simulink model "mcb_microchip_pmsm_foc_sensorless_PIC32MK1024MCF"  (R2023b)
settings: Solver=FixedStepDiscrete  StartTime=0.0  StopTime=5  FixedStep=Ts  RelTol=1e-3  EnableMultiTasking=on
InitFcn:
  | mcb_microchip_pmsm_foc_sensorless_pic32mk_data
values from neighbouring files (symbols this model uses):
  PI_params = mcb.internal.SetControllerParameters(pmsm,inverter,PU_System,T_pwm,2*Ts,Ts_speed)    [mcb_microchip_pmsm_foc_sensorless_pic32mk_data.m]
  PU_System = mcb_SetPUSystem(pmsm,inverter)    [mcb_microchip_pmsm_foc_sensorless_pic32mk_data.m]
  PWM_frequency = 12e3    (= 12000)    [mcb_microchip_pmsm_foc_sensorless_pic32mk_data.m]
  Ts = T_pwm    (= 8.33333333333e-05)    [mcb_microchip_pmsm_foc_sensorless_pic32mk_data.m]
  Ts_motor = T_pwm    (= 8.33333333333e-05)    [mcb_microchip_pmsm_foc_sensorless_pic32mk_data.m]
  Ts_simulink = T_pwm    (= 8.33333333333e-05)    [mcb_microchip_pmsm_foc_sensorless_pic32mk_data.m]
  Ts_speed = 1e-3    (= 0.001)    [mcb_microchip_pmsm_foc_sensorless_pic32mk_data.m]
  Vd_Ref_openLoop_PU = 0.15    [mcb_microchip_pmsm_foc_sensorless_pic32mk_data.m]
undefined symbols (not defined in the file or in its folder): A0, A11, A4, AN24, AN9, B6, B9, C8, DiscIntNeverNeededParam, inverter, Pin, pmsm, Timer
libraries: simulink x16, MCHP_Blockset x12, mcbcontrolslib x10, slpidlib x3, mcbpositiondecoderlib x2, mcbplantlib x1, autolibpmsmexterior x1
(part 2 of 3)

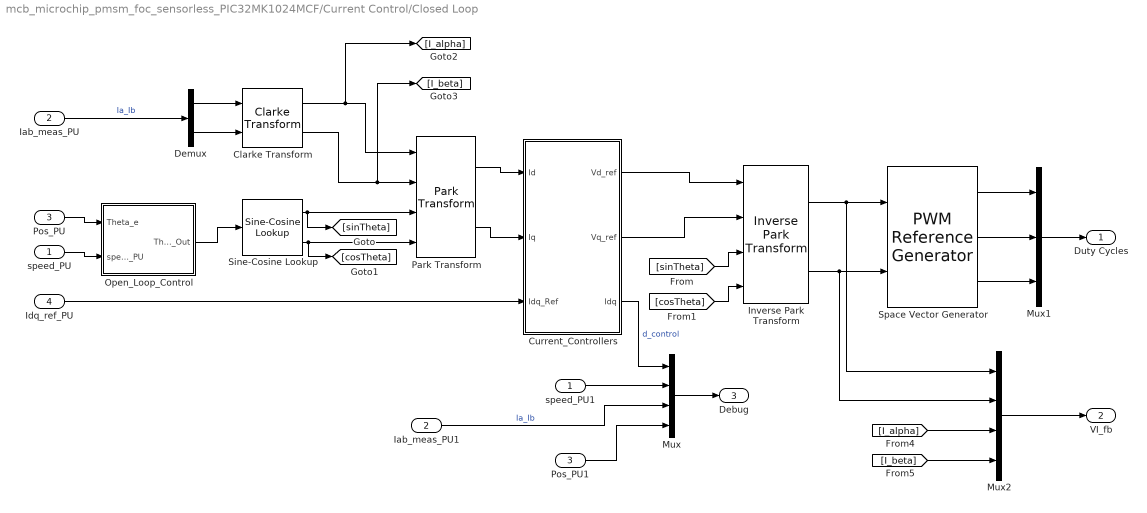
== system mcb_microchip_pmsm_foc_sensorless_PIC32MK1024MCF/Current Control/Closed Loop ==
  speed_PU : Inport
  Iab_meas_PU : Inport  Port=2
  Pos_PU : Inport  Port=3
  Idq_ref_PU : Inport  Port=4
  Clarke Transform : mcbcontrolslib/Clarke Transform  VariantControl=Variant2  PhaseInput=Two inputs  EnPowerInv=off
  Current_Controllers : Subsystem
  Demux : Demux  Outputs=2
  Iab_meas_PU1 : InportShadow  Port=2
  Inverse Park Transform : mcbcontrolslib/Inverse Park Transform  PhaseInput=Two inputs  AxisAlignment=D-axis  ThetaInput=Sine and Cosine electrical position  AngleInput=Per-unit  N_points=1024
  Mux : Mux
  Mux1 : Mux  Inputs=3
  Mux2 : Mux
  Open_Loop_Control : Subsystem
  Park Transform : mcbcontrolslib/Park Transform  PhaseInput=Two inputs  AxisAlignment=D-axis  ThetaInput=Sine and Cosine electrical position  AngleInput=Per-unit  N_points=1024
  Pos_PU1 : InportShadow  Port=3
  Sine-Cosine Lookup : mcbcontrolslib/Sine-Cosine Lookup  AngleInput=Per-unit  N_points=1024
  Space Vector Generator : mcbcontrolslib/PWM Reference Generator  inSignal=Valphabeta  modType=SVM: space vector modulation
  speed_PU1 : InportShadow
  Duty Cycles : Outport  VectorParamsAs1DForOutWhenUnconnected=off
  VI_fb : Outport  Port=2  VectorParamsAs1DForOutWhenUnconnected=off
  Debug : Outport  Port=3  VectorParamsAs1DForOutWhenUnconnected=off
  wires:
  Current_Controllers/1(Vd_ref) -> Inverse Park Transform/1
  [cosTheta] -> Inverse Park Transform/4
  [I_beta] -> Mux2/4
  Inverse Park Transform/2 -> Space Vector Generator/2, Mux2/2
  Inverse Park Transform/1 -> Space Vector Generator/1, Mux2/1
  [sinTheta] -> Inverse Park Transform/3
  Mux2/1 -> VI_fb/1
  Clarke Transform/1 -> [I_alpha], Park Transform/1
  Current_Controllers/2(Vq_ref) -> Inverse Park Transform/2
  Clarke Transform/2 -> [I_beta], Park Transform/2
  Sine-Cosine Lookup/1 -> [sinTheta], Park Transform/3
  [I_alpha] -> Mux2/3
  Space Vector Generator/1 -> Mux1/1
  Space Vector Generator/3 -> Mux1/3
  Mux1/1 -> Duty Cycles/1
  Sine-Cosine Lookup/2 -> Park Transform/4, [cosTheta]
  Space Vector Generator/2 -> Mux1/2
  Park Transform/1 -> Current_Controllers/1(Id)
  Park Transform/2 -> Current_Controllers/2(Iq)
  Demux/1 -> Clarke Transform/1
  Demux/2 -> Clarke Transform/2
  Iab_meas_PU/1 -> Demux/1  "Ia_Ib"
  Idq_ref_PU/1 -> Current_Controllers/3(Idq_Ref)
  Pos_PU/1 -> Open_Loop_Control/1(Theta_e)
  Open_Loop_Control/1(Theta_Out) -> Sine-Cosine Lookup/1
  speed_PU/1 -> Open_Loop_Control/2(speed_PU)
  speed_PU1/1 -> Mux/2
  Current_Controllers/3(Idq) -> Mux/1  "d_control"
  Mux/1 -> Debug/1
  Iab_meas_PU1/1 -> Mux/3  "Ia_Ib"
  Pos_PU1/1 -> Mux/4

== system mcb_microchip_pmsm_foc_sensorless_PIC32MK1024MCF/Current Control/HW Inputs ==
  Sim : Inport
  Sensor Driver Blocks (codegen) : Subsystem  VariantControl=(codegen)
  Sensor Driver Blocks (sim) : Subsystem  VariantControl=(sim)
  Iab_ADC : Outport

== system mcb_microchip_pmsm_foc_sensorless_PIC32MK1024MCF/Current Control/Input Scaling ==
  note: Current Measurements
  Iab_ADC : Inport
  VI_fb : Inport  Port=2
  Calculate Phase Currents : Subsystem
  Calculate position and speed : Subsystem
  speed_PU : Outport
  Iab_meas_PU : Outport  Port=2
  Pos_PU : Outport  Port=3
  wires:
  Calculate Phase Currents/1(Iab_meas_PU) -> Iab_meas_PU/1  "Iab_fb_PU"
  Iab_ADC/1 -> Calculate Phase Currents/1(Iab_ADC)
  Calculate position and speed/2(speed_PU) -> speed_PU/1
  Calculate position and speed/1(Pos_PU) -> Pos_PU/1
  VI_fb/1 -> Calculate position and speed/1(VI_fb)

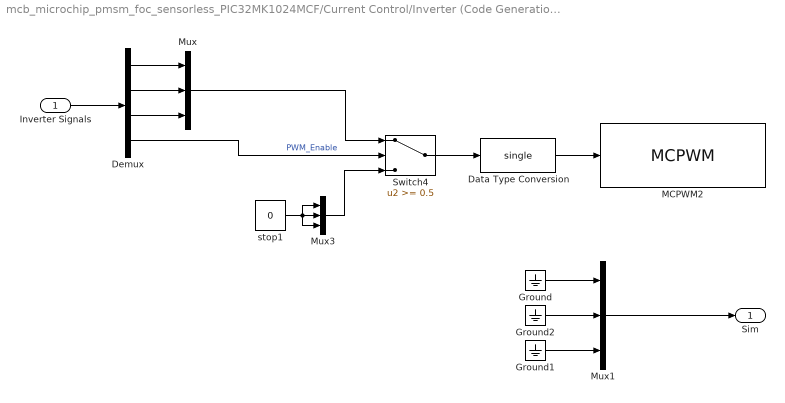
== system mcb_microchip_pmsm_foc_sensorless_PIC32MK1024MCF/Current Control/Inverter (Code Generation) ==
  Inverter Signals : Inport
  Data Type Conversion : DataTypeConversion  OutDataTypeStr=single  SaturateOnIntegerOverflow=off  RndMeth=Floor
  Demux : Demux
  Ground : Ground
  Ground1 : Ground
  Ground2 : Ground
  MCPWM2 : MCHP_Blockset/PWM IO/MCPWM  Priority=-2000  PWMx_ECAM_ITB=Independant - Center aligned - Symetric  PWMx_MTBS=Primary master timer  PWM_ClockResolution=Dynamic Options  PWM_ClockResolution_TXT=auto  MaxPeriod_s=Ts  InitPeriode_s=Ts  InitDutyCycleP_s=10e-6  InitDutyCycleS_s=10e-6  InitPhase_s=-1  SampleTime=Ts  S_INPUT=[-1]  S_INPUT_Size=[3]  S_OUTPUT=[]  S_OUTPUT_Size=[]  S_ListCustomDatatype=S.S_ListCustomDatatype={};  MCHP_USER_INTERRUPTS=0  evalin_ws=PWM1max=MCHP_Fun.Hex2num('40B3880000000000');PWM2max=MCHP_Fun.Hex2num('40B3880000000000');PWM3max=MCHP_Fun.Hex2num('40B3880000000000');  MCHP_PORT={PWMH1 }{PWMH1}32:4:B14;{PWMH2 }{PWMH2}32:4:B12;{PWMH3 }{PWMH3}32:4:B10;{PWML1}{PWML1}32:4:B15;{PWML2}{PWML2}32:4:B13;{PWML3}{PWML3}32:4:B11;{PWM FLT15}{FLT15}32:0:B4;  MCHP_MASTERLINK=mcb_microchip_pmsm_foc_sensorless_PIC32MK/Configurations/Microchip Master  MCHP_CRC=3937595  PWMx_PMOD=Complementary  PWM1_HL=PWMxH & PWMxL output enabled  PWM1_swap=off  PWM1H_pol=off  PWM1L_pol=off  PWM2_HL=PWMxH & PWMxL output enabled  PWM2_swap=off  PWM2H_pol=off  PWM2L_pol=off  PWM3_HL=PWMxH & PWMxL output enabled  PWM3_swap=off  PWM3H_pol=off  PWM3L_pol=off  PWM4_HL=not used  PWM4_swap=off  PWM4H_pol=off  PWM4L_pol=off  PWM5_HL=not used  PWM5_swap=off  PWM5H_pol=off  PWM5L_pol=off  PWM6_HL=not used  PWM6_swap=off  PWM6H_pol=off  PWM6L_pol=off  PWM7_HL=not used  PWM7_swap=off  PWM7H_pol=off  PWM7L_pol=off  PWM8_HL=not used  PWM8_swap=off  PWM8H_pol=off  PWM8L_pol=off  PWM9_HL=not used  PWM9_swap=off  PWM9H_pol=off  PWM9L_pol=off  PWM10_HL=not used  PWM10_swap=off  PWM10H_pol=off  PWM10L_pol=off  PWM11_HL=not used  PWM11_swap=off  PWM11H_pol=off  PWM11L_pol=off  PWM12_HL=not used  PWM12_swap=off  PWM12H_pol=off  PWM12L_pol=off  Init_SEVTCMP_SSEVTCMP=-1  Init_TRIGx_STRIGx_1=[1.8e-6 ,-1]  Init_TRIGx_STRIGx_2=[-1 -1]  Init_TRIGx_STRIGx_3=[-1 -1]  Init_TRIGx_STRIGx_4=[-1 -1]  Init_TRIGx_STRIGx_5=[-1 -1]  Init_TRIGx_STRIGx_6=[-1 -1]  Init_TRIGx_STRIGx_7=[-1 -1]  Init_TRIGx_STRIGx_8=[-1 -1]  Init_TRIGx_STRIGx_9=[-1 -1]  Init_TRIGx_STRIGx_10=[-1 -1]  Init_TRIGx_STRIGx_11=[-1 -1]  Init_TRIGx_STRIGx_12=[-1 -1]  TRIG_DualTriggerMode=Primary Trigger to ADC is independant  BlockInput_VectorScalar=Vectors (grouped by function)  BlockInput_Period=Not a block input  BlockInput_DutyCycle=a Floating Point input within range [-1 1]  BlockInput_PhaseShift=Not a block input  BlockInput_SEVTCMP=Not a block input  BlockInput_TRIGx=Not a block input  BlockInput_DeadTime=Not a block input  BlockOutput_FaultDisabled=off  BlockOutput_Fault=off  DTC=Positive dead time (ensure period of time with PWM_H and PWM_L disasserted)  FLTSRC1_DTCMP=Dynamic Options  FLTSRC1_DTCMP_TXT="FLT6 / E13 / Pin[42]  -  Active HIGH"  FLTSRC2_DTCMP=Dynamic Options  FLTSRC2_DTCMP_TXT="FLT6 / E13 / Pin[42]  -  Active LOW"  FLTSRC3_DTCMP=Dynamic Options  FLTSRC3_DTCMP_TXT="FLT8 / E15 / Pin[44]  -  Active LOW"  FLTSRC4_DTCMP=Dynamic Options  FLTSRC4_DTCMP_TXT="FLT3 / C2 / Pin[34]  -  Active HIGH"  FLTSRC5_DTCMP=Dynamic Options  FLTSRC5_DTCMP_TXT="FLT3 / C2 / Pin[34]  -  Active HIGH"  FLTSRC6_DTCMP=Dynamic Options  FLTSRC6_DTCMP_TXT="FLT3 / C2 / Pin[34]  -  Active HIGH"  FLTSRC7_DTCMP=Dynamic Options  FLTSRC7_DTCMP_TXT="FLT3 / C2 / Pin[34]  -  Active HIGH"  FLTSRC8_DTCMP=Dynamic Options  FLTSRC8_DTCMP_TXT="FLT3 / C2 / Pin[34]  -  Active HIGH"  FLTSRC9_DTCMP=Dynamic Options  FLTSRC9_DTCMP_TXT="FLT3 / C2 / Pin[34]  -  Active HIGH"  FLTSRC10_DTCMP=Dynamic Options  FLTSRC10_DTCMP_TXT="FLT3 / C2 / Pin[34]  -  Active HIGH"  FLTSRC11_DTCMP=Dynamic Options  FLTSRC11_DTCMP_TXT="FLT3 / C2 / Pin[34]  -  Active HIGH"  FLTSRC12_DTCMP=Dynamic Options  FLTSRC12_DTCMP_TXT="FLT3 / C2 / Pin[34]  -  Active HIGH"  DeadTime_s=2e-6  DeadTimeAlt_s=2e-6  DeadTimeComp_s=0  FLTMODx=Force PWM output for current cycle. Enable PWM on next cycle  FLTSRCx=Dynamic Options  FLTSRCx_TXT="FLT15 / B4 / Pin[50]  -  Active LOW"  FLTDATx=PWM H/L -> 00  CLMODx=Disabled  CLSRCx=Dynamic Options  CLSRCx_TXT="FLT8 / E15 / Pin[44]  -  Active LOW"  CLDATx=PWM H/L -> 00  FLTLEBENx=off  CLLEBENx=off  LeadEdgeBlkPer_s=5e-7  PHRx=off  PHFx=off  PLRx=off  PLFx=off
      settings: SourceProductName=MPLAB Device Blocks for Simulink
  Mux : Mux  Inputs=3
  Mux1 : Mux  Inputs=3
  Mux3 : Mux  Inputs=3
  Switch4 : Switch  Threshold=0.5  RndMeth=Simplest  SaturateOnIntegerOverflow=off  InputSameDT=off
  stop1 : Constant  Value=0  OutDataTypeStr=dataType
  Sim : Outport  VectorParamsAs1DForOutWhenUnconnected=off
  wires:
  Inverter Signals/1 -> Demux/1
  Ground/1 -> Mux1/1
  Ground1/1 -> Mux1/3
  Ground2/1 -> Mux1/2
  Mux1/1 -> Sim/1
  Demux/1 -> Mux/1
  Demux/2 -> Mux/2
  Demux/3 -> Mux/3
  Switch4/1 -> Data Type Conversion/1
  Data Type Conversion/1 -> MCPWM2/1
  stop1/1 -> Mux3/3, Mux3/2, Mux3/1
  Mux/1 -> Switch4/1
  Mux3/1 -> Switch4/3
  Demux/4 -> Switch4/2  "PWM_Enable"

== system mcb_microchip_pmsm_foc_sensorless_PIC32MK1024MCF/Current Control/Inverter (Simulation) ==
  Inverter Signals : Inport
  Data Type Duplicate : DataTypeDuplicate
  Demux : Demux
  Mux : Mux  Inputs=3
  Mux2 : Mux  Inputs=3
  Subsystem : Subsystem
  Switch1 : Switch  Threshold=0.5  RndMeth=Simplest  SaturateOnIntegerOverflow=off  InputSameDT=off
  stop : Constant  Value=0  OutDataTypeStr=Inherit: Inherit via back propagation
  Sim : Outport  VectorParamsAs1DForOutWhenUnconnected=off
  wires:
  stop/1 -> Data Type Duplicate/2, Mux2/1, Mux2/3, Mux2/2
  Mux2/1 -> Switch1/3
  Switch1/1 -> Sim/1
  Inverter Signals/1 -> Demux/1
  Demux/4 -> Switch1/2  "PWM Enable"
  Mux/1 -> Subsystem/1(In1), Data Type Duplicate/1  "PWM Duty Cycles"
  Demux/1 -> Mux/1
  Demux/2 -> Mux/2
  Demux/3 -> Mux/3
  Subsystem/1(PWM_Duty_Cycles) -> Switch1/1  "test"

== system mcb_microchip_pmsm_foc_sensorless_PIC32MK1024MCF/Current Control/Output Scaling ==
  PWM_Duty : Inport
  Constant2 : Constant  Value=0  OutDataTypeStr=Inherit: Inherit via back propagation
  Data Type Conversion : DataTypeConversion  OutDataTypeStr=dataType  SaturateOnIntegerOverflow=off  RndMeth=Floor
  Enable : DataStoreRead  DataStoreName=Enable  IndexOptions=Index vector (dialog)  Indices=1  OutputSizes=1
  Mode Selector : Subsystem
  Mux1 : Mux  Inputs=3
  Switch for Current offset calibration : Switch  Criteria=u2 ~= 0  Threshold=250  SaturateOnIntegerOverflow=off  InputSameDT=off
  PWM_Duty_Cycles : Outport
  PWM_Enable : Outport  Port=2
  wires:
  Data Type Conversion/1 -> PWM_Enable/1
  Enable/1 -> Data Type Conversion/1
  PWM_Duty/1 -> Switch for Current offset calibration/3
  Mode Selector/1(CurrentOffsetEn) -> Switch for Current offset calibration/2
  Mux1/1 -> Switch for Current offset calibration/1
  Constant2/1 -> Mux1/3, Mux1/2, Mux1/1
  Switch for Current offset calibration/1 -> PWM_Duty_Cycles/1

== system mcb_microchip_pmsm_foc_sensorless_PIC32MK1024MCF/Inverter and Motor - Plant Model/Plant Model ==
  Duty_Cycles : Inport
  Inverter and Motor (codegen) : Subsystem  VariantControl=(codegen)
  Inverter and Motor (sim) : Subsystem  VariantControl=(sim)
  Feedbacks_sim : Outport  VectorParamsAs1DForOutWhenUnconnected=off

== system mcb_microchip_pmsm_foc_sensorless_PIC32MK1024MCF/Serial Receive/CodeGen ==
  Data Store Write1 : DataStoreWrite  DataStoreName=Debug_signals  IndexOptions=Index vector (dialog)  Indices=1  OutputSizes=1
  Data Type Conversion : DataTypeConversion  OutDataTypeStr=uint16  SaturateOnIntegerOverflow=off  RndMeth=Floor
  Subsystem : Subsystem
  Subsystem1 : Subsystem
  UART Rx : MCHP_Blockset/BUS UART/UART Rx  UART_REF=2  Flag_Out=on  Rx_Size_popup=User defined  Rx_Size=1  S_Rx_Size=1  Split=Read all received char  SplitChar=10  OutputDefault_popup=do nothing (end of output vector will be undefined)  OutputDefault=-2  ORDERING=None  SampleTime=.001  MCHP_MASTERLINK=mcb_microchip_pmsm_foc_sensorless_PIC32MK/Configurations/Microchip Master  MCHP_COMPILED_INFO="CompiledSampleTime= [0.0010000000000000000208   0 ];CompiledInportDataTypes=[    ];CompiledInportDataWidth=[];"
      settings: SourceProductName=MPLAB Device Blocks for Simulink
  SpeedRef : Outport
  Enable : Outport  Port=2
  wires:
  UART Rx/1 -> Data Type Conversion/1
  Subsystem/3(Debug Signal Selection) -> Data Store Write1/1
  UART Rx/2 -> Subsystem1/1(In1)
  Subsystem/2(Enable) -> Enable/1
  Subsystem/1(SpeedRef) -> SpeedRef/1
  Subsystem1/2(Data out) -> Subsystem/1(In1)
  Subsystem1/1(NewData) -> Subsystem/Enable
  Data Type Conversion/1 -> Subsystem1/Enable

== system mcb_microchip_pmsm_foc_sensorless_PIC32MK1024MCF/Serial Receive/Sim ==
  Data Type Conversion1 : DataTypeConversion  OutDataTypeStr=dataType  RndMeth=Simplest  SaturateOnIntegerOverflow=off
  Data Type Conversion2 : DataTypeConversion  OutDataTypeStr=boolean  RndMeth=Simplest  SaturateOnIntegerOverflow=off
  Gain : Gain  Gain=1/PU_System.N_base  RndMeth=Simplest  OutDataTypeStr=Inherit: Same as input
  Speed Ref [RPM] : Step  Time=3.5  Before=0.2 * PU_System.N_base  After=0.8 * PU_System.N_base  OutDataTypeStr=single  SampleTime=0.001
  Step1 : Step  OutDataTypeStr=single  SampleTime=0.001
  SpeedRef : Outport
  Enable : Outport  Port=2
  wires:
  Speed Ref [RPM]/1 -> Gain/1
  Data Type Conversion1/1 -> SpeedRef/1
  Step1/1 -> Data Type Conversion2/1
  Data Type Conversion2/1 -> Enable/1
  Gain/1 -> Data Type Conversion1/1

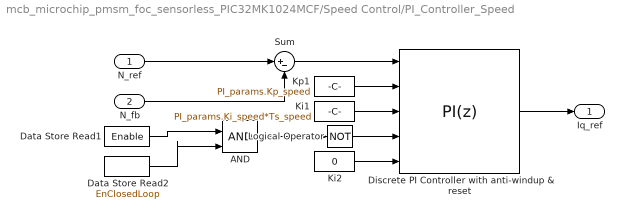
== system mcb_microchip_pmsm_foc_sensorless_PIC32MK1024MCF/Speed Control/PI_Controller_Speed ==
  N_ref : Inport
  N_fb : Inport  Port=2
  AND : Logic  IconShape=distinctive  AllPortsSameDT=off  OutDataTypeStr=boolean
  Data Store Read2 : DataStoreRead  DataStoreName=EnClosedLoop  IndexOptions=Index vector (dialog)  Indices=1  OutputSizes=1
  Data Store Read1 : DataStoreRead  DataStoreName=Enable  IndexOptions=Index vector (dialog)  Indices=1  OutputSizes=1
  Discrete PI Controller with anti-windup & reset : slpidlib/PID Controller  Controller=PI  Form=Parallel  TimeDomain=Discrete-time  UseExternalTs=off  SampleTime=-1  IntegratorMethod=Forward Euler  FilterMethod=Forward Euler  ControllerParametersSource=external  P=1  I=1  UseKiTs=on  D=0  N=100  UseFilter=on  TunerSelectOption=Transfer Function Based (PID Tuner App)  InitialConditionSource=external  InitialConditionForIntegrator=0  InitialConditionForFilter=0  DifferentiatorICPrevScaledInput=0  ExternalReset=level  TrackingMode=off  Kt=1  LimitOutput=on  SatLimitsSource=internal  UpperSaturationLimit=1  LowerSaturationLimit=-1  LinearizeAsGain=on  AntiWindupMode=clamping  Kb=1  LimitIntegrator=off  UpperIntegratorSaturationLimit=inf  LowerIntegratorSaturationLimit=-inf  RndMeth=Simplest  POutMin=[]  POutMax=[]  IOutMin=[]  IOutMax=[]  DOutMin=[]  DOutMax=[]  NOutMin=[]  NOutMax=[]  SumOutMin=[]  SumOutMax=[]  SaturationOutDataTypeStr=Inherit: Inherit via back propagation  SaturationOutMin=[]  SaturationOutMax=[]  PParamMin=[]  PParamMax=[]  IParamMin=[]  IParamMax=[]  DParamMin=[]  DParamMax=[]  NParamMin=[]  NParamMax=[]  KbParamMin=[]  KbParamMax=[]  KtParamMin=[]  KtParamMax=[]  KbOutMin=[]  KbOutMax=[]  KtOutMin=[]  KtOutMax=[]  IntegratorOutMin=[]  IntegratorOutMax=[]  FilterOutMin=[]  FilterOutMax=[]  SumI1OutMin=[]  SumI1OutMax=[]  SumI2OutMin=[]  SumI2OutMax=[]  SumI3OutMin=[]  SumI3OutMax=[]  SumI4OutMin=[]  SumI4OutMax=[]  SumDOutMin=[]  SumDOutMax=[]  DifferentiatorOutMin=[]  DifferentiatorOutMax=[]  FilterDiffOutCoefMin=[]  FilterDiffOutCoefMax=[]  ReciprocalOutMin=[]  ReciprocalOutMax=[]  SumDenOutMin=[]  SumDenOutMax=[]  SumNumOutMin=[]  SumNumOutMax=[]  DivideOutMin=[]  DivideOutMax=[]  UdiffTsProdOutMin=[]  UdiffTsProdOutMax=[]  NTsProdOutMin=[]  NTsProdOutMax=[]  UintegralTsProdOutMin=[]  UintegralTsProdOutMax=[]  UngainTsProdOutMin=[]  UngainTsProdOutMax=[]  ClampingZeroOutDataTypeStr=Inherit: Inherit via back propagation  ClampingZeroOutMin=[]  ClampingZeroOutMax=[]  FilterDenConstantOutDataTypeStr=Inherit: Inherit via back propagation  FilterDenConstantOutMin=[]  FilterDenConstantOutMax=[]  PCopyOutDataTypeStr=Inherit: Inherit via back propagation  PCopyOutMin=[]  PCopyOutMax=[]  NCopyOutDataTypeStr=Inherit: Inherit via back propagation  NCopyOutMin=[]  NCopyOutMax=[]  IntegratorContinuousStateAttributes=''  IntegratorStateMustResolveToSignalObject=off  IntegratorRTWStateStorageClass=Auto  FilterContinuousStateAttributes=''  FilterStateMustResolveToSignalObject=off  FilterRTWStateStorageClass=Auto  ParallelPVariant=ExternalParameters  IdealPVariant=Disabled  IVariant=ExternalParameters  DVariant=Disabled  IntegratorVariant=Discrete  SatVariant=Enabled  AWVariant=DiscClampingParallel  PCopyVariant=Disabled  TRVariant=Disabled  FdbkBlocksVariant=Forward  IdealPFdbkVariant=Disabled  SatFdbkVariant=Disabled  DerivativeFilterVariant=Disabled  NVariant=Disabled  NCopyVariant=Disabled_SignalSpec  FilterICVariant=Disabled  IntegratorICVariant=ExternalICs  ExternalResetVariant=ExternalReset  TRSumVariant=Passthrough  SumFdbkVariant=Disabled  SumVariant=Sum_PI  TsampFilterVariant=InternalTs  TsampNgainVariant=Passthrough  TsampIntegralVariant=Disabled_SignalSpec  ExternalSaturationOutDataTypeStr=Inherit: Same as second input
      settings: LibrarySourceBlock=mcbcontrolslib/PI Controller
  Ki1 : Constant  Value=PI_params.Ki_speed*Ts_speed  OutDataTypeStr=dataType  SampleTime=-1
  Ki2 : Constant  Value=0  OutDataTypeStr=dataType  SampleTime=-1
  Kp1 : Constant  Value=PI_params.Kp_speed  OutDataTypeStr=dataType  SampleTime=-1
  Logical Operator : Logic  Operator=NOT  IconShape=distinctive  AllPortsSameDT=off  OutDataTypeStr=boolean
  Sum : Sum  Inputs=|+-  OutDataTypeStr=Inherit: Same as first input
  Iq_ref : Outport  VectorParamsAs1DForOutWhenUnconnected=off
  wires:
  Discrete PI Controller with anti-windup & reset/1 -> Iq_ref/1
  Ki1/1 -> Discrete PI Controller with anti-windup & reset/3
  Kp1/1 -> Discrete PI Controller with anti-windup & reset/2
  N_fb/1 -> Sum/2
  N_ref/1 -> Sum/1
  Sum/1 -> Discrete PI Controller with anti-windup & reset/1
  Logical Operator/1 -> Discrete PI Controller with anti-windup & reset/4
  Ki2/1 -> Discrete PI Controller with anti-windup & reset/5
  Data Store Read1/1 -> AND/1
  Data Store Read2/1 -> AND/2
  AND/1 -> Logical Operator/1

== system mcb_microchip_pmsm_foc_sensorless_PIC32MK1024MCF/Speed Control/Speed_Ref_Selector ==
  Speed_Ref : Inport
  Constant : Constant  Value=0.1  OutDataTypeStr=dataType
  Constant1 : Constant  Value=-0.1  OutDataTypeStr=dataType
  Data Store Read : DataStoreRead  DataStoreName=Speed_ref  IndexOptions=Index vector (dialog)  Indices=1  OutputSizes=1
  Data Store Read1 : DataStoreRead  DataStoreName=EnClosedLoop  IndexOptions=Index vector (dialog)  Indices=1  OutputSizes=1
  IIR Filter : mcbcontrolslib/IIR Filter  VariantControl=Low Pass Filter  VariantSelect=Low-pass  Filter_constant=0.001*(Ts_speed/Ts)  advancedSettings=off  Ts=50e-6  cutOff_freq=38.6611
  Switch : Switch  Criteria=u2 > Threshold  SaturateOnIntegerOverflow=off  InputSameDT=off
  Switch1 : Switch  Criteria=u2 > Threshold  SaturateOnIntegerOverflow=off  InputSameDT=off
  Speed_Ref1 : Outport
  wires:
  IIR Filter/1 -> Speed_Ref1/1  "Speed_Ref"
  Data Store Read1/1 -> Switch/2
  Switch/1 -> IIR Filter/1  "Speed_Ref"
  Constant/1 -> Switch1/1
  Data Store Read/1 -> Switch1/2
  Switch1/1 -> Switch/3
  Speed_Ref/1 -> Switch/1
  Constant1/1 -> Switch1/3

== system mcb_microchip_pmsm_foc_sensorless_PIC32MK1024MCF/Subsystem2/Data ==
  Data : Inport
  Action Port : ActionPort  ActionPortLabel=else
  UART Tx : MCHP_Blockset/BUS UART/UART Tx  UART_REF=2  ORDERING=None  AllOrNothing=off  SampleTime=-1  MCHP_MASTERLINK=mcb_microchip_pmsm_foc_sensorless_PIC32MK/Configurations/Microchip Master  NSend_Input=off  UART_String=off  NSend_Output=off
      settings: SourceProductName=MPLAB Device Blocks for Simulink
  wires:
  Data/1 -> UART Tx/1

== system mcb_microchip_pmsm_foc_sensorless_PIC32MK1024MCF/Subsystem2/End ==
  Data : Inport
  Action Port : ActionPort  ActionPortLabel=elseif(u1 == 29)
  Mux : Mux  Inputs=2
  Start : Constant  Value=hex2dec('45')  OutDataTypeStr=uint8
  UART Tx : MCHP_Blockset/BUS UART/UART Tx  UART_REF=2  ORDERING=None  AllOrNothing=off  SampleTime=-1  MCHP_MASTERLINK=mcb_microchip_pmsm_foc_sensorless_PIC32MK/Configurations/Microchip Master  NSend_Input=off  UART_String=off  NSend_Output=off
      settings: SourceProductName=MPLAB Device Blocks for Simulink
  wires:
  Start/1 -> Mux/2
  Data/1 -> Mux/1
  Mux/1 -> UART Tx/1

== system mcb_microchip_pmsm_foc_sensorless_PIC32MK1024MCF/Subsystem2/Start ==
  Data : Inport
  Action Port : ActionPort  ActionPortLabel=if(u1 == 0)
  End : Constant  Value=hex2dec('53')  OutDataTypeStr=uint8
  Mux : Mux  Inputs=2
  UART Tx : MCHP_Blockset/BUS UART/UART Tx  UART_REF=2  ORDERING=None  AllOrNothing=off  SampleTime=-1  MCHP_MASTERLINK=mcb_microchip_pmsm_foc_sensorless_PIC32MK/Configurations/Microchip Master  NSend_Input=off  UART_String=off  NSend_Output=off
      settings: SourceProductName=MPLAB Device Blocks for Simulink
  wires:
  End/1 -> Mux/1
  Data/1 -> Mux/2
  Mux/1 -> UART Tx/1

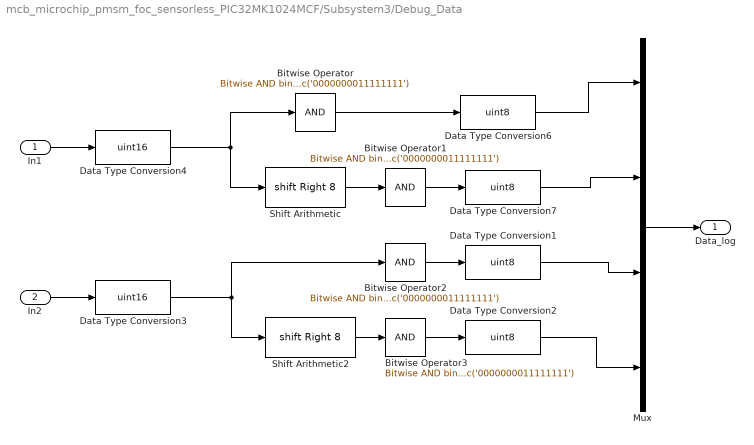
== system mcb_microchip_pmsm_foc_sensorless_PIC32MK1024MCF/Subsystem3/Debug_Data ==
  In1 : Inport
  In2 : Inport  Port=2
  Bitwise Operator{,1..3} (4 alike) : simulink/Logic and Bit Operations/Bitwise Operator  logicop=AND  UseBitMask=on  BitMask=bin2dec('0000000011111111')  BitMaskRealWorld=Stored Integer
  Data Type Conversion{1..2,6..7} (4 alike) : DataTypeConversion  OutDataTypeStr=uint8  RndMeth=Simplest  SaturateOnIntegerOverflow=off
  Data Type Conversion3 : DataTypeConversion  OutDataTypeStr=uint16  ConvertRealWorld=Stored Integer (SI)  RndMeth=Simplest  SaturateOnIntegerOverflow=off
  Data Type Conversion4 : DataTypeConversion  OutDataTypeStr=uint16  ConvertRealWorld=Stored Integer (SI)  RndMeth=Simplest  SaturateOnIntegerOverflow=off
  Mux : Mux
  Shift Arithmetic : ArithShift  BitShiftNumber=8  BitShiftDirection=Right
  Shift Arithmetic2 : ArithShift  BitShiftNumber=8  BitShiftDirection=Right
  Data_log : Outport
  wires:
  Mux/1 -> Data_log/1
  In1/1 -> Data Type Conversion4/1
  Data Type Conversion4/1 -> Shift Arithmetic/1, Bitwise Operator/1
  Data Type Conversion6/1 -> Mux/1
  Data Type Conversion7/1 -> Mux/2
  Bitwise Operator2/1 -> Data Type Conversion1/1
  Data Type Conversion1/1 -> Mux/3
  Bitwise Operator/1 -> Data Type Conversion6/1
  Shift Arithmetic/1 -> Bitwise Operator1/1
  Data Type Conversion2/1 -> Mux/4
  Bitwise Operator1/1 -> Data Type Conversion7/1
  Shift Arithmetic2/1 -> Bitwise Operator3/1
  Bitwise Operator3/1 -> Data Type Conversion2/1
  Data Type Conversion3/1 -> Shift Arithmetic2/1, Bitwise Operator2/1
  In2/1 -> Data Type Conversion3/1

== system mcb_microchip_pmsm_foc_sensorless_PIC32MK1024MCF/Current Control/Closed Loop/Current_Controllers ==
  Id : Inport
  Iq : Inport  Port=2
  Idq_Ref : Inport  Port=3
  DQ Limiter : mcbcontrolslib/DQ Limiter  satMethodInputType=Specify via dialog  satMethodSelected=D-Q equivalence  satLimitInputType=Specify via dialog  Vmax=1
  Demux : Demux  Outputs=2
  Mux : Mux
  PI_Controller_Id : Subsystem
  PI_Controller_Iq : Subsystem
  Terminator : Terminator
  Vd_ref : Outport  VectorParamsAs1DForOutWhenUnconnected=off
  Vq_ref : Outport  Port=2  VectorParamsAs1DForOutWhenUnconnected=off
  Idq : Outport  Port=3  VectorParamsAs1DForOutWhenUnconnected=off
  wires:
  Iq/1 -> Mux/4, PI_Controller_Iq/2(I_fb)  "Iq_fb"
  PI_Controller_Id/1(V_ref) -> DQ Limiter/1
  Id/1 -> PI_Controller_Id/2(I_fb), Mux/2  "Id_fb"
  Demux/1 -> PI_Controller_Id/1(I_ref), Mux/1  "Id_Ref"
  Demux/2 -> Mux/3, PI_Controller_Iq/1(I_ref)  "Iq_Ref"
  DQ Limiter/1 -> Vd_ref/1
  DQ Limiter/2 -> Vq_ref/1
  PI_Controller_Iq/1(V_ref) -> DQ Limiter/2
  DQ Limiter/3 -> Terminator/1
  Idq_Ref/1 -> Demux/1
  Mux/1 -> Idq/1

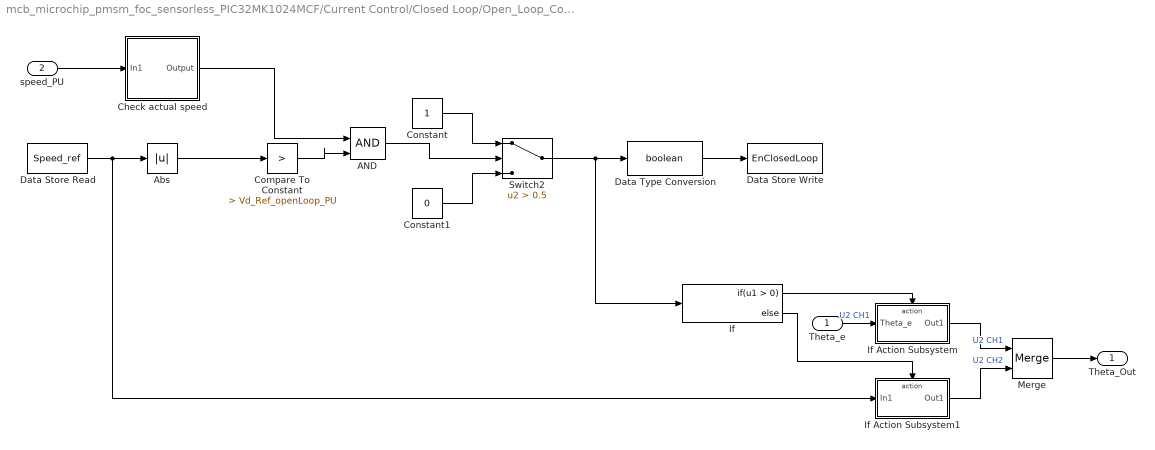
== system mcb_microchip_pmsm_foc_sensorless_PIC32MK1024MCF/Current Control/Closed Loop/Open_Loop_Control ==
  Theta_e : Inport
  speed_PU : Inport  Port=2
  AND : Logic  IconShape=distinctive  AllPortsSameDT=off  OutDataTypeStr=boolean
  Abs : Abs  SaturateOnIntegerOverflow=off
  Check actual speed : Subsystem
  Compare To Constant : simulink/Logic and Bit Operations/Compare To Constant  relop=>  const=Vd_Ref_openLoop_PU  OutDataTypeStr=boolean
  Constant : Constant  OutDataTypeStr=uint16
  Constant1 : Constant  Value=0  OutDataTypeStr=uint16
  Data Store Read : DataStoreRead  DataStoreName=Speed_ref  IndexOptions=Index vector (dialog)  Indices=1  OutputSizes=1
  Data Store Write : DataStoreWrite  DataStoreName=EnClosedLoop  IndexOptions=Index vector (dialog)  Indices=1  OutputSizes=1
  Data Type Conversion : DataTypeConversion  OutDataTypeStr=boolean  RndMeth=Simplest  SaturateOnIntegerOverflow=off
  If : If
  If Action Subsystem : Subsystem  TreatAsAtomicUnit=on
  If Action Subsystem1 : Subsystem  TreatAsAtomicUnit=on
  Merge : Merge
  Switch2 : Switch  Criteria=u2 > Threshold  Threshold=0.5  SaturateOnIntegerOverflow=off  InputSameDT=off
  Theta_Out : Outport
  wires:
  Theta_e/1 -> If Action Subsystem/1(Theta_e)  "U2 CH1"
  If/2 -> If Action Subsystem1/Action
  Switch2/1 -> If/1, Data Type Conversion/1
  If Action Subsystem1/1(Out1) -> Merge/2  "U2 CH2"
  Data Type Conversion/1 -> Data Store Write/1
  Check actual speed/1(Output) -> AND/1
  If Action Subsystem/1(Out1) -> Merge/1  "U2 CH1"
  If/1 -> If Action Subsystem/Action
  Abs/1 -> Compare To Constant/1
  Merge/1 -> Theta_Out/1
  speed_PU/1 -> Check actual speed/1(In1)
  Data Store Read/1 -> If Action Subsystem1/1(In1), Abs/1
  Constant1/1 -> Switch2/3
  Compare To Constant/1 -> AND/2
  AND/1 -> Switch2/2
  Constant/1 -> Switch2/1

== system mcb_microchip_pmsm_foc_sensorless_PIC32MK1024MCF/Current Control/HW Inputs/Sensor Driver Blocks (codegen) ==
  Sim : Inport
  ADC PIC32 High Speed SAR1 : MCHP_Blockset/Analog IO/ADC PIC32 High Speed SAR  Priority=-5000  ADC_VrefH=AVdd (default)  ADC_VrefL=AVss (default)  ADC_FRACT=Integer (right aligned)  DMA_Size=Single trigger - (no DMA)  ADC_Synchronisation=Triggered by custom source  ADC_Trig=Dynamic Options  ADC_Trig_TXT=PWM1 trigger  ADC_TrigTimeStep=off  ADC_TrigInfo=0  SampleTime=Ts  S_INPUT=[]  S_INPUT_Size=[]  S_OUTPUT="[4  4]"  S_OUTPUT_Size="[1  1]"  S_ListCustomDatatype=S.S_ListCustomDatatype={};  MCHP_USER_INTERRUPTS={AD1D0}{ADC0Data}{ADC Data 0 Ready}{VectorName(ADC_DATA0_VECTOR) Priority(-1) Config_BitSet(ADCGIRQEN1bits.AGIEN0) RegisterReadClear(ADCDATA0)};{AD1D4}{ADC4Data}{ADC Data 4 Ready}{VectorName(ADC_DATA4_VECTOR) Priority(-1) Config_BitSet(ADCGIRQEN1bits.AGIEN4) RegisterReadClear(ADCDATA4)};  MCHP_PORT={Analog Input 24}{AN24}15:2:A4;{Analog Input 9}{AN9}15:2:A11;  MCHP_MASTERLINK=mcb_microchip_pmsm_foc_sensorless_PIC32MK/Configurations/Microchip Master  MCHP_CRC=3308460  ADC_Info=Total Time = 450(ns)  ADC0_pin=Dynamic Options  ADC0_pin_TXT=AN24 / A4 / Pin[51]  ADC0_R=< 200 Ohm  ADC0_res=12 bits  ADC0_signed=unsigned 16 bits  ADC0_FILTER=No Oversampling  ADC0_FILTER_nSamples=256 samples  ADC0_STRGEN=End sampling and start conversion  ADC0_SSAMPEN=on  ADC0_Info=tSmp_min=100(ns) x 0 = 0(s) ; tConv=433.33(ns) x 1 = 433.33(ns) ; TOTAL=450(ns)  ADC1_pin=Dynamic Options  ADC1_pin_TXT=Not used  ADC1_R=< 200 Ohm  ADC1_res=12 bits  ADC1_signed=signed 16 bits  ADC1_FILTER=No Oversampling  ADC1_FILTER_nSamples=256 samples  ADC1_STRGEN=End sampling and start conversion  ADC1_SSAMPEN=on  ADC1_Info=tSmp_min=33.333(ns) x -1 = -33.333(ns) ; tConv=166.67(ns) x 0 = 0(s) ; TOTAL=0(s)  ADC2_pin=Dynamic Options  ADC2_pin_TXT=Not used  ADC2_R=< 200 Ohm  ADC2_res=12 bits  ADC2_signed=signed 16 bits  ADC2_FILTER=No Oversampling  ADC2_FILTER_nSamples=256 samples  ADC2_STRGEN=End sampling and start conversion  ADC2_SSAMPEN=on  ADC2_Info=tSmp_min=33.333(ns) x -1 = -33.333(ns) ; tConv=166.67(ns) x 0 = 0(s) ; TOTAL=0(s)  ADC3_pin=Dynamic Options  ADC3_pin_TXT=Not used  ADC3_R=< 200 Ohm  ADC3_res=12 bits  ADC3_signed=unsigned 16 bits  ADC3_FILTER=No Oversampling  ADC3_FILTER_nSamples=256 samples  ADC3_STRGEN=End sampling and start conversion  ADC3_SSAMPEN=on  ADC3_Info=tSmp_min=33.333(ns) x -1 = -33.333(ns) ; tConv=166.67(ns) x 0 = 0(s) ; TOTAL=0(s)  ADC4_pin=Dynamic Options  ADC4_pin_TXT=AN9 / A11 / Pin[21]  ADC4_R=< 200 Ohm  ADC4_res=12 bits  ADC4_signed=unsigned 16 bits  ADC4_FILTER=No Oversampling  ADC4_FILTER_nSamples=256 samples  ADC4_STRGEN=End sampling and start conversion  ADC4_SSAMPEN=on  ADC4_Info=tSmp_min=100(ns) x 0 = 0(s) ; tConv=433.33(ns) x 1 = 433.33(ns) ; TOTAL=450(ns)  ADC5_pin=Dynamic Options  ADC5_pin_TXT=Not used  ADC5_R=< 200 Ohm  ADC5_res=12 bits  ADC5_signed=unsigned 16 bits  ADC5_FILTER=No Oversampling  ADC5_FILTER_nSamples=256 samples  ADC5_STRGEN=End sampling and start conversion  ADC5_SSAMPEN=off  ADC5_Info=tSmp_min=33.333(ns) x -1 = -33.333(ns) ; tConv=166.67(ns) x 0 = 0(s) ; TOTAL=0(s)  ADC6_pin=Dynamic Options  ADC6_pin_TXT=Not used  ADC6_R=< 200 Ohm  ADC6_res=12 bits  ADC6_signed=unsigned 16 bits  ADC6_FILTER=Burst convert of n samples are Summed  ADC6_FILTER_nSamples=256 samples  ADC6_STRGEN=End sampling and start conversion  ADC6_SSAMPEN=on  ADC6_Info=tSmp_min=33.333(ns) x -1 = -33.333(ns) ; tConv=166.67(ns) x 0 = 0(s) ; TOTAL=0(s)  ADC7_R=< 200 Ohm  ADC7_res=12 bits  ADC7_AN0=Not used  ADC7_AN1=Not used  ADC7_AN2=Not used  ADC7_AN3=Not used  ADC7_AN4=Not used  ADC7_AN5=Not used  ADC7_AN6=Not used  ADC7_AN7=Not used  ADC7_AN8=Not used  ADC7_AN9=Not used  ADC7_AN10=Not used  ADC7_AN11=Not used  ADC7_AN12=Not used  ADC7_AN13=Not used  ADC7_AN14=Not used  ADC7_AN15=Not used  ADC7_AN16=Not used  ADC7_AN17=Not used  ADC7_AN18=Not used  ADC7_AN19=Not used  ADC7_AN20=Not used  ADC7_AN21=Not used  ADC7_AN22=Not used  ADC7_AN23=Not used  ADC7_AN24=Not used  ADC7_AN25=Not used  ADC7_AN26=Not used  ADC7_AN27=Not used  ADC7_AN28=Not used  ADC7_AN29=Not used  ADC7_AN30=Not used  ADC7_AN31=Not used  ADC7_AN32=Not used  ADC7_AN33=Not used  ADC7_AN34=Not used  ADC7_AN35=Not used  ADC7_AN36=Not used  ADC7_AN37=Not used  ADC7_AN38=Not used  ADC7_AN39=Not used  ADC7_AN40=Not used  ADC7_AN41=Not used  ADC7_AN42=Not used  ADC7_AN43=Not used  ADC7_AN44=Not used  ADC7_AN45=Not used  ADC7_AN46=Not used  ADC7_AN47=Not used  ADC7_AN48=Not used  ADC7_AN49=Not used  ADC7_AN50=Not used  ADC7_AN51=Not used  ADC7_AN52=Not used  ADC7_AN53=Not used  ADC7_AN54=Not used  ADC7_AN55=Not used  ADC7_AN56=Not used  ADC7_AN57=Not used  ADC7_AN58=Not used  ADC7_AN59=Not used  ADC7_AN60=Not used  ADC7_AN61=Not used  ADC7_AN62=Not used  ADC7_AN63=Not used  CTMU_Temp=Not used  Vbat=Not used  IVref=Not used  IVTemp=Not used
      settings: SourceProductName=MPLAB Device Blocks for Simulink
  Mux : Mux  Inputs=2
  Terminator : Terminator
  Iab_ADC : Outport
  wires:
  Sim/1 -> Terminator/1
  Mux/1 -> Iab_ADC/1
  ADC PIC32 High Speed SAR1/1 -> Mux/1
  ADC PIC32 High Speed SAR1/2 -> Mux/2

== system mcb_microchip_pmsm_foc_sensorless_PIC32MK1024MCF/Current Control/HW Inputs/Sensor Driver Blocks (sim) ==
  Sim : Inport
  Iab_ADC : Outport
  wires:
  Sim/1 -> Iab_ADC/1

== system mcb_microchip_pmsm_foc_sensorless_PIC32MK1024MCF/Current Control/Input Scaling/Calculate Phase Currents ==
  Iab_ADC : Inport
  Add : Sum  Inputs=-+
  Data Store Read2 : DataStoreRead  DataStoreName=EnCurOffset  IndexOptions=Index vector (dialog)  Indices=1  OutputSizes=1
  Data Type Conversion : DataTypeConversion  OutDataTypeStr=int32  ConvertRealWorld=Stored Integer (SI)  SaturateOnIntegerOverflow=off  RndMeth=Floor
  Data Type Conversion1 : DataTypeConversion  OutDataTypeStr=dataType  SaturateOnIntegerOverflow=off  RndMeth=Floor
  Gain1 : Gain  Gain=1/2048  OutDataTypeStr=Inherit: Same as input  ParamDataTypeStr=Inherit: Same as input
  Offset : Subsystem
  Iab_meas_PU : Outport  VectorParamsAs1DForOutWhenUnconnected=off
  wires:
  Add/1 -> Data Type Conversion1/1
  Data Type Conversion1/1 -> Gain1/1
  Data Store Read2/1 -> Offset/Enable
  Data Type Conversion/1 -> Add/1, Offset/1(Iab)
  Offset/1(Offset) -> Add/2
  Iab_ADC/1 -> Data Type Conversion/1  "U2 CH1"
  Gain1/1 -> Iab_meas_PU/1  "U2 CH1"

== system mcb_microchip_pmsm_foc_sensorless_PIC32MK1024MCF/Current Control/Input Scaling/Calculate position and speed ==
  VI_fb : Inport
  Demux : Demux  Outputs=2
  Sliding Mode Observer : Subsystem
  Pos_PU : Outport
  speed_PU : Outport  Port=2
  wires:
  VI_fb/1 -> Sliding Mode Observer/1(InputSignals)
  Demux/1 -> Pos_PU/1
  Demux/2 -> speed_PU/1
  Sliding Mode Observer/1(Position/Speed) -> Demux/1

== system mcb_microchip_pmsm_foc_sensorless_PIC32MK1024MCF/Current Control/Inverter (Simulation)/Subsystem ==
  In1 : Inport
  Constant : Constant  Value=0.5  OutDataTypeStr=dataType
  Gain : Gain  Gain=0.5  OutDataTypeStr=Inherit: Same as input
  Sum : Sum  Inputs=|++
  PWM_Duty_Cycles : Outport
  wires:
  Gain/1 -> Sum/1
  Constant/1 -> Sum/2
  In1/1 -> Gain/1
  Sum/1 -> PWM_Duty_Cycles/1  "PWM_Duty_Cycles"

== system mcb_microchip_pmsm_foc_sensorless_PIC32MK1024MCF/Current Control/Output Scaling/Mode Selector ==
  Delay : Delay  DelayLength=1
  NOT : Logic  Operator=NOT  IconShape=distinctive  AllPortsSameDT=off  OutDataTypeStr=boolean
  Subsystem1 : Subsystem
  Up Counter : Subsystem
  CurrentOffsetEn : Outport
  wires:
  Up Counter/1(Count) -> Subsystem1/1(Count)
  Delay/1 -> NOT/1
  NOT/1 -> Up Counter/Enable
  Subsystem1/2(EnClosedLoop) -> Delay/1
  Subsystem1/1(Current Offset) -> CurrentOffsetEn/1

== system mcb_microchip_pmsm_foc_sensorless_PIC32MK1024MCF/Inverter and Motor - Plant Model/Plant Model/Inverter and Motor (codegen) ==
  Duty_Cycles : Inport
  Ground : Ground
  Terminator : Terminator
  Feedbacks_sim : Outport  VectorParamsAs1DForOutWhenUnconnected=off
  wires:
  Duty_Cycles/1 -> Terminator/1
  Ground/1 -> Feedbacks_sim/1

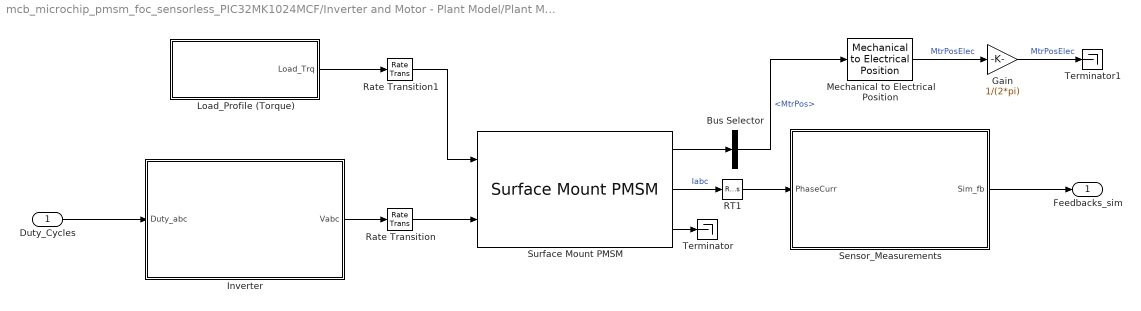
== system mcb_microchip_pmsm_foc_sensorless_PIC32MK1024MCF/Inverter and Motor - Plant Model/Plant Model/Inverter and Motor (sim) ==
  Duty_Cycles : Inport
  Bus Selector : BusSelector  OutputSignals=MtrPos
  Gain : Gain  Gain=1/(2*pi)  OutDataTypeStr=Inherit: Same as input
  Inverter : Subsystem
  Load_Profile (Torque) : Subsystem
  Mechanical to Electrical Position : mcbpositiondecoderlib/Mechanical to Electrical Position  PolePairsInputType=Specify via dialog  NrPP=pmsm.p  selectedRange=Radians  MechOfstInputType=Specify via dialog  mechOffsetIn=0  maxAngleIn=2*pi  InputDataType=single  VariantSelect=floating-point
  RT1 : RateTransition  Deterministic=off  OutPortSampleTime=Ts_simulink
  Rate Transition : RateTransition  Deterministic=off  OutPortSampleTime=Ts_motor
  Rate Transition1 : RateTransition  Deterministic=off  OutPortSampleTime=Ts_motor
  Sensor_Measurements : Subsystem
  Surface Mount PMSM : autolibpmsmexterior/Surface Mount PMSM  port_config=Torque  sim_type=Discrete  Ts=Ts_motor  FilePath=surfacepmsm_motordata.m  P=pmsm.p  Rs=pmsm.Rs + inverter.R_board  Ldq_=pmsm.Ld  KConstText=Permanent flux linkage constant (lambda_pm):  lambda_pm=pmsm.FluxPM  Ke=159.9771  Kt=1.323  mechanical=[pmsm.J, pmsm.B, 0]  idq0=[0 0]  theta_init=0  omega_init=0  KConst=pmsm.FluxPM  lambda_pm_calc=pmsm.FluxPM  RefBlkName='autolibpmsmexterior/Surface Mount PMSM'  aMode=5  Ldq="[0.00078136  0.00078136]"
  Terminator : Terminator
  Terminator1 : Terminator
  Feedbacks_sim : Outport  VectorParamsAs1DForOutWhenUnconnected=off
  wires:
  Inverter/1(Vabc) -> Rate Transition/1
  Surface Mount PMSM/2 -> RT1/1  "Iabc"
  Sensor_Measurements/1(Sim_fb) -> Feedbacks_sim/1
  Surface Mount PMSM/3 -> Terminator/1
  Load_Profile (Torque)/1(Load_Trq) -> Rate Transition1/1
  Duty_Cycles/1 -> Inverter/1(Duty_abc)
  Rate Transition/1 -> Surface Mount PMSM/2
  Rate Transition1/1 -> Surface Mount PMSM/1
  RT1/1 -> Sensor_Measurements/1(PhaseCurr)
  Gain/1 -> Terminator1/1  "MtrPosElec"
  Mechanical to Electrical Position/1 -> Gain/1  "MtrPosElec"
  Bus Selector/1 -> Mechanical to Electrical Position/1  "<MtrPos>"
  Surface Mount PMSM/1 -> Bus Selector/1

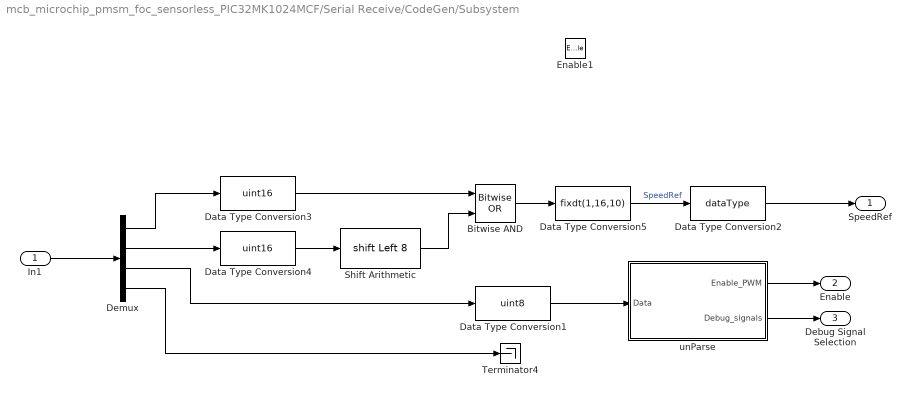
== system mcb_microchip_pmsm_foc_sensorless_PIC32MK1024MCF/Serial Receive/CodeGen/Subsystem ==
  In1 : Inport
  Enable1 : EnablePort
  Bitwise AND : simulink/Logic and Bit Operations/Bitwise Operator  logicop=OR  UseBitMask=off  NumInputPorts=2  BitMask=bin2dec('11011001')  BitMaskRealWorld=Stored Integer
  Data Type Conversion1 : DataTypeConversion  OutDataTypeStr=uint8  RndMeth=Simplest  SaturateOnIntegerOverflow=off
  Data Type Conversion2 : DataTypeConversion  OutDataTypeStr=dataType  RndMeth=Simplest  SaturateOnIntegerOverflow=off
  Data Type Conversion3 : DataTypeConversion  OutDataTypeStr=uint16  RndMeth=Simplest  SaturateOnIntegerOverflow=off
  Data Type Conversion4 : DataTypeConversion  OutDataTypeStr=uint16  RndMeth=Simplest  SaturateOnIntegerOverflow=off
  Data Type Conversion5 : DataTypeConversion  OutDataTypeStr=fixdt(1,16,10)  ConvertRealWorld=Stored Integer (SI)  SaturateOnIntegerOverflow=off
  Demux : Demux
  Shift Arithmetic : ArithShift  BitShiftNumber=8  BitShiftDirection=Left
  Terminator4 : Terminator
  unParse : Subsystem
  SpeedRef : Outport
  Enable : Outport  Port=2
  Debug Signal Selection : Outport  Port=3
  wires:
  Data Type Conversion4/1 -> Shift Arithmetic/1
  Data Type Conversion3/1 -> Bitwise AND/1
  In1/1 -> Demux/1
  unParse/2(Debug_signals) -> Debug Signal Selection/1
  Data Type Conversion2/1 -> SpeedRef/1
  Demux/3 -> Data Type Conversion1/1
  Bitwise AND/1 -> Data Type Conversion5/1
  unParse/1(Enable_PWM) -> Enable/1
  Data Type Conversion1/1 -> unParse/1(Data)
  Demux/2 -> Data Type Conversion4/1
  Demux/4 -> Terminator4/1
  Shift Arithmetic/1 -> Bitwise AND/2
  Data Type Conversion5/1 -> Data Type Conversion2/1  "SpeedRef"
  Demux/1 -> Data Type Conversion3/1

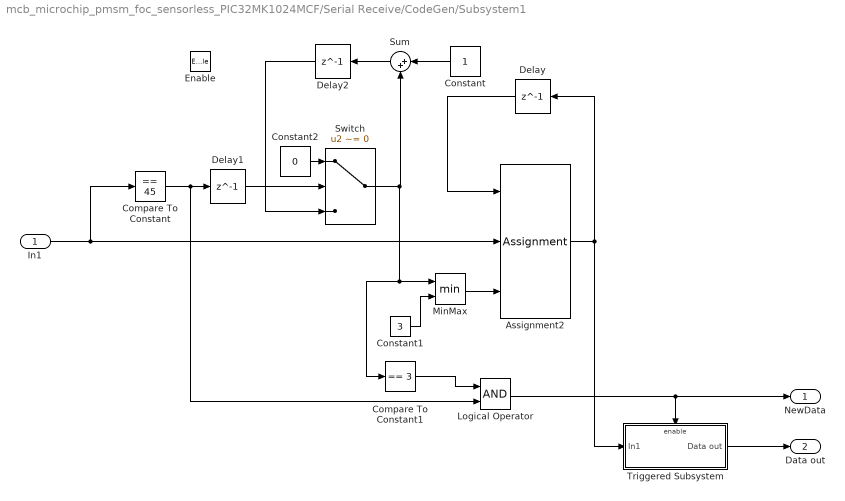
== system mcb_microchip_pmsm_foc_sensorless_PIC32MK1024MCF/Serial Receive/CodeGen/Subsystem1 ==
  In1 : Inport
  Enable : EnablePort
  Assignment2 : Assignment  IndexMode=Zero-based  DiagnosticForDimensions=Warning  IndexOptions=Starting index (port)  Indices=1  OutputSizes=1
  Compare To Constant : simulink/Logic and Bit Operations/Compare To Constant  relop===  const=45  OutDataTypeStr=boolean
  Compare To Constant1 : simulink/Logic and Bit Operations/Compare To Constant  relop===  const=3  OutDataTypeStr=boolean
  Constant : Constant  OutDataTypeStr=uint16  SampleTime=-1
  Constant1 : Constant  Value=3  OutDataTypeStr=uint16  SampleTime=-1
  Constant2 : Constant  Value=0  OutDataTypeStr=uint16  SampleTime=-1
  Delay : Delay  DelayLength=1  InitialCondition=[0 0 0 0]
  Delay1 : Delay  DelayLength=1  InitialCondition=0
  Delay2 : Delay  DelayLength=1  InitialCondition=0
  Logical Operator : Logic  AllPortsSameDT=off  OutDataTypeStr=boolean
  MinMax : MinMax  Inputs=2
  Sum : Sum  Inputs=|++
  Switch : Switch  Criteria=u2 ~= 0  SaturateOnIntegerOverflow=off  InputSameDT=off
  Triggered Subsystem : Subsystem  TreatAsAtomicUnit=on
  NewData : Outport  OutputWhenDisabled=reset  InitialOutput=0
  Data out : Outport  Port=2
  wires:
  Logical Operator/1 -> Triggered Subsystem/Enable, NewData/1
  Triggered Subsystem/1(Data out) -> Data out/1
  Constant2/1 -> Switch/1
  Delay1/1 -> Switch/2
  Switch/1 -> MinMax/1, Compare To Constant1/1, Sum/2
  Sum/1 -> Delay2/1
  MinMax/1 -> Assignment2/3
  Constant1/1 -> MinMax/2
  Constant/1 -> Sum/1
  In1/1 -> Assignment2/2, Compare To Constant/1
  Compare To Constant1/1 -> Logical Operator/1
  Compare To Constant/1 -> Delay1/1, Logical Operator/2
  Delay2/1 -> Switch/3
  Delay/1 -> Assignment2/1
  Assignment2/1 -> Delay/1, Triggered Subsystem/1(In1)

== system mcb_microchip_pmsm_foc_sensorless_PIC32MK1024MCF/Current Control/Closed Loop/Current_Controllers/PI_Controller_Id ==
  I_ref : Inport
  I_fb : Inport  Port=2
  Data Store Read1 : DataStoreRead  DataStoreName=EnClosedLoop  IndexOptions=Index vector (dialog)  Indices=1  OutputSizes=1
  Discrete PI Controller with anti-windup & reset : slpidlib/PID Controller  Controller=PI  Form=Parallel  TimeDomain=Discrete-time  UseExternalTs=off  SampleTime=-1  IntegratorMethod=Forward Euler  FilterMethod=Forward Euler  ControllerParametersSource=external  P=1  I=1  UseKiTs=on  D=0  N=100  UseFilter=on  TunerSelectOption=Transfer Function Based (PID Tuner App)  InitialConditionSource=external  InitialConditionForIntegrator=0  InitialConditionForFilter=0  DifferentiatorICPrevScaledInput=0  ExternalReset=level  TrackingMode=off  Kt=1  LimitOutput=on  SatLimitsSource=internal  UpperSaturationLimit=1  LowerSaturationLimit=-1  LinearizeAsGain=on  AntiWindupMode=clamping  Kb=1  LimitIntegrator=off  UpperIntegratorSaturationLimit=inf  LowerIntegratorSaturationLimit=-inf  RndMeth=Simplest  POutMin=[]  POutMax=[]  IOutMin=[]  IOutMax=[]  DOutMin=[]  DOutMax=[]  NOutMin=[]  NOutMax=[]  SumOutMin=[]  SumOutMax=[]  SaturationOutDataTypeStr=Inherit: Inherit via back propagation  SaturationOutMin=[]  SaturationOutMax=[]  PParamMin=[]  PParamMax=[]  IParamMin=[]  IParamMax=[]  DParamMin=[]  DParamMax=[]  NParamMin=[]  NParamMax=[]  KbParamMin=[]  KbParamMax=[]  KtParamMin=[]  KtParamMax=[]  KbOutMin=[]  KbOutMax=[]  KtOutMin=[]  KtOutMax=[]  IntegratorOutMin=[]  IntegratorOutMax=[]  FilterOutMin=[]  FilterOutMax=[]  SumI1OutMin=[]  SumI1OutMax=[]  SumI2OutMin=[]  SumI2OutMax=[]  SumI3OutMin=[]  SumI3OutMax=[]  SumI4OutMin=[]  SumI4OutMax=[]  SumDOutMin=[]  SumDOutMax=[]  DifferentiatorOutMin=[]  DifferentiatorOutMax=[]  FilterDiffOutCoefMin=[]  FilterDiffOutCoefMax=[]  ReciprocalOutMin=[]  ReciprocalOutMax=[]  SumDenOutMin=[]  SumDenOutMax=[]  SumNumOutMin=[]  SumNumOutMax=[]  DivideOutMin=[]  DivideOutMax=[]  UdiffTsProdOutMin=[]  UdiffTsProdOutMax=[]  NTsProdOutMin=[]  NTsProdOutMax=[]  UintegralTsProdOutMin=[]  UintegralTsProdOutMax=[]  UngainTsProdOutMin=[]  UngainTsProdOutMax=[]  ClampingZeroOutDataTypeStr=Inherit: Inherit via back propagation  ClampingZeroOutMin=[]  ClampingZeroOutMax=[]  FilterDenConstantOutDataTypeStr=Inherit: Inherit via back propagation  FilterDenConstantOutMin=[]  FilterDenConstantOutMax=[]  PCopyOutDataTypeStr=Inherit: Inherit via back propagation  PCopyOutMin=[]  PCopyOutMax=[]  NCopyOutDataTypeStr=Inherit: Inherit via back propagation  NCopyOutMin=[]  NCopyOutMax=[]  IntegratorContinuousStateAttributes=''  IntegratorStateMustResolveToSignalObject=off  IntegratorRTWStateStorageClass=Auto  FilterContinuousStateAttributes=''  FilterStateMustResolveToSignalObject=off  FilterRTWStateStorageClass=Auto  ParallelPVariant=ExternalParameters  IdealPVariant=Disabled  IVariant=ExternalParameters  DVariant=Disabled  IntegratorVariant=Discrete  SatVariant=Enabled  AWVariant=DiscClampingParallel  PCopyVariant=Disabled  TRVariant=Disabled  FdbkBlocksVariant=Forward  IdealPFdbkVariant=Disabled  SatFdbkVariant=Disabled  DerivativeFilterVariant=Disabled  NVariant=Disabled  NCopyVariant=Disabled_SignalSpec  FilterICVariant=Disabled  IntegratorICVariant=ExternalICs  ExternalResetVariant=ExternalReset  TRSumVariant=Passthrough  SumFdbkVariant=Disabled  SumVariant=Sum_PI  TsampFilterVariant=InternalTs  TsampNgainVariant=Passthrough  TsampIntegralVariant=Disabled_SignalSpec  ExternalSaturationOutDataTypeStr=Inherit: Same as second input
      settings: LibrarySourceBlock=mcbcontrolslib/PI Controller
  Ki : Constant  Value=PI_params.Ki_i*Ts  OutDataTypeStr=dataType  SampleTime=-1
  Kp : Constant  Value=PI_params.Kp_i  OutDataTypeStr=dataType  SampleTime=-1
  Logical Operator : Logic  Operator=NOT  IconShape=distinctive  AllPortsSameDT=off  OutDataTypeStr=boolean
  Sum : Sum  Inputs=|+-  OutDataTypeStr=Inherit: Same as first input
  Switch : Switch  Criteria=u2 ~= 0  RndMeth=Simplest  SaturateOnIntegerOverflow=off  InputSameDT=off
  Unit Delay : UnitDelay  SampleTime=-1  HasFrameUpgradeWarning=on
  Vd_OpenLoop : Constant  Value=Vd_Ref_openLoop_PU  OutDataTypeStr=dataType  SampleTime=-1
  V_ref : Outport  VectorParamsAs1DForOutWhenUnconnected=off
  wires:
  Switch/1 -> V_ref/1, Unit Delay/1
  I_fb/1 -> Sum/2
  Sum/1 -> Discrete PI Controller with anti-windup & reset/1
  Kp/1 -> Discrete PI Controller with anti-windup & reset/2
  I_ref/1 -> Sum/1
  Ki/1 -> Discrete PI Controller with anti-windup & reset/3
  Logical Operator/1 -> Discrete PI Controller with anti-windup & reset/4
  Unit Delay/1 -> Discrete PI Controller with anti-windup & reset/5
  Discrete PI Controller with anti-windup & reset/1 -> Switch/1
  Vd_OpenLoop/1 -> Switch/3
  Data Store Read1/1 -> Logical Operator/1, Switch/2
